simulink model "PhysModel013"  (R2016b)
settings: Solver=VariableStepAuto  StartTime=0.0  StopTime=10.0  RelTol=1e-3
libraries: simulink x2
settings Model: Creator=gwb15193  LastModifiedBy=gwb15193
settings DataIOCC: ReturnWorkspaceOutputs=on
settings SFSimCC: SimUseLocalCustomCode=on
settings RTWCC: RTWUseLocalCustomCode=on

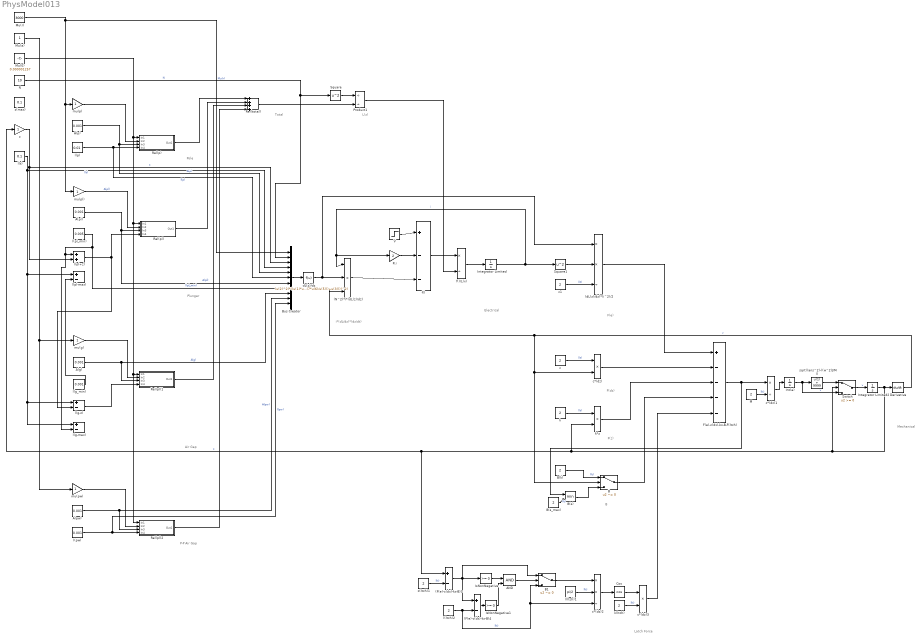
== system PhysModel013 ==
  note: Latch Force
  note: F(dz)
  note: F(e)
  note: i*(dL/dz)*(dz/dt)
  note: Mechanical
  note: Electrical
  note: Total
  note: Pole
  note: Plunger
  note: Air Gap
  note: P-P Air Gap
  note: L(z)
  note: F(z)
  note: B
  (F(e)-c(dx)-kx-B)3 : Sum  Inputs=+-
  (F(e)-c(dx)-kx-B)4 : Sum  Inputs=+-
  (N^2)*i*(dL(z)/dz) : Product  Inputs=***
  (dL(z)/dz)*(i^2)/2 : Product  Inputs=**/
  A(g) : Constant  Value=0.001
  A(p) : Constant  Value=0.001
  A(pl) : Constant  Value=0.001
  A(pw) : Constant  Value=0.001
  AND : Logic  IconShape=distinctive  AllPortsSameDT=off  OutDataTypeStr=boolean
  B : Switch  Criteria=u2 ~= 0
  B(k) : Constant  Value=2
  B(s) : MinMax  Inputs=2
  B(s_max) : Constant  Value=2
  B1 : Switch  Criteria=u2 ~= 0
  Bus Creator : BusCreator  Inputs=11
  Cos : Trigonometry  Operator=cos
  Derivative : Derivative
  F(e)-c(dx)-kx-B-F(ltch) : Sum  Inputs=+----
  Int(a) : Integrator  LimitOutput=on  UpperSaturationLimit=1  LowerSaturationLimit=0
  Integrator Limited : Integrator  LimitOutput=on  UpperSaturationLimit=1  LowerSaturationLimit=0
  Integrator Limited2 : Integrator  LimitOutput=on  UpperSaturationLimit=1  LowerSaturationLimit=0
  IsNonNegative : simulink/Logic and Bit Operations/Compare To Zero  relop=>=  OutDataTypeStr=boolean
  IsNonNegative1 : simulink/Logic and Bit Operations/Compare To Zero  relop=>=  OutDataTypeStr=boolean
  M : Constant  Value=2
  Mu(0) : Constant  Value=0.000001257
  Mu(a) : Constant
  Mu(r) : Constant  Value=3000
  N : Constant  Value=10
  Product1 : Product  Inputs=//
  R.i : Gain  Gain=2
  Rel(p) : Subsystem
  Rel(pl) : Subsystem
  Rel(pl)1 : Subsystem
  Rel(pl)2 : Subsystem
  Rel(total) : Sum  Inputs=++++
  Square : Math  Operator=square  SaturateOnIntegerOverflow=on
  Square1 : Math  Operator=square  SaturateOnIntegerOverflow=on
  Switch : Switch
  V : Step  Time=10  After=10  SampleTime=0
  c : Constant  Value=2
  c*(dz) : Product  Inputs=**
  c*(dz)1 : Product  Inputs=*/
  c*(dz)2 : Product  Inputs=**/
  c*(dz)3 : Product  Inputs=**
  c1 : Constant  Value=2
  dL(z)/dz : Fcn  Expr=(u(2)^2)*((u(1)*u(7)*u(9))*(u(1)*u(7)-u(9))/(((u(1)*u(7))*(u(4)-u(8)+(u(9)*u(11)/u(10))-u(3)))+(u(9)*(u(8)+(u(7*u(6)/u(5)))+u(3))))^2)
  f() : Sum  Inputs=+--
  f()/L(x) : Product  Inputs=*/
  k : Constant  Value=2
  k(ltch) : Constant  Value=2
  k*z : Product  Inputs=**
  l(g-max) : Sum  Inputs=+-
  l(g-z) : Sum  Inputs=+-
  l(g_min) : Constant  Value=0.001
  l(ltch)1 : Constant  Value=pi/2
  l(ltch)2 : Constant  Value=2
  l(p) : Constant  Value=0.01
  l(pl+z) : Sum
  l(pl-max) : Sum  Inputs=+-
  l(pl_min) : Constant  Value=0.005
  l(pw) : Constant  Value=0.001
  l(t) : Constant  Value=0.1
  mu(g) : Gain
  mu(p) : Gain
  mu(pl) : Gain
  mu(pw) : Gain
  sqrt((ans^2)-((w^2)J/M)) : Fcn  Expr=u(1) + 9999
  z : Gain
  z(ltch)1 : Constant  Value=2
  z(max) : Constant  Value=0.1
  wires:
  l(p)/1 -> Bus Creator/6, Rel(p)/4(In4)  "l(p)"
  A(p)/1 -> Bus Creator/5, Rel(p)/3(In3)  "A(p)"
  l(pl+z)/1 -> l(g-z)/2, Rel(pl)/4(In4)
  A(pl)/1 -> Rel(pl)/3(In3), Bus Creator/7  "A(pl)"
  mu(p)/1 -> Rel(p)/2(In2)
  mu(g)/1 -> Rel(pl)1/2(In2)
  A(g)/1 -> Bus Creator/9, Rel(pl)1/3(In3)  "A(g)"
  l(g-z)/1 -> Rel(pl)1/4(In4)
  l(g_min)/1 -> l(pl-max)/2
  A(pw)/1 -> Bus Creator/10, Rel(pl)2/3(In3)  "A(pw)"
  Mu(r)/1 -> Bus Creator/1, mu(pl)/1, mu(p)/1  "Mu(r)"
  l(pw)/1 -> Bus Creator/11, Rel(pl)2/4(In4)  "l(pw)"
  mu(pw)/1 -> Rel(pl)2/2(In2)
  Mu(0)/1 -> Rel(pl)2/1(In1), Rel(pl)1/1(In1), Rel(pl)/1(In1), Rel(p)/1(In1)
  Rel(p)/1(Out1) -> Rel(total)/1
  Rel(pl)/1(Out1) -> Rel(total)/2
  Rel(pl)1/1(Out1) -> Rel(total)/3
  Rel(pl)2/1(Out1) -> Rel(total)/4
  Mu(a)/1 -> mu(pw)/1, mu(g)/1
  l(pl_min)/1 -> Bus Creator/8, l(g-max)/2, l(pl+z)/1  "l(pl_min)"
  z/1 -> l(pl+z)/2, Bus Creator/3  "z"
  Square/1 -> Product1/1
  N/1 -> Bus Creator/2, Square/1  "N"
  Rel(total)/1 -> Product1/2
  f()/L(x)/1 -> Integrator Limited/1
  R.i/1 -> f()/2
  V/1 -> f()/1
  f()/1 -> f()/L(x)/1
  (N^2)*i*(dL(z)/dz)/1 -> f()/3
  Product1/1 -> f()/L(x)/2
  sqrt((ans^2)-((w^2)J/M))/1 -> Switch/1
  Switch/1 -> Integrator Limited2/1  "v"
  Integrator Limited/1 -> R.i/1, (N^2)*i*(dL(z)/dz)/1, Square1/1  "i"
  Int(a)/1 -> sqrt((ans^2)-((w^2)J/M))/1, Switch/3  "v"
  Derivative/1 -> (N^2)*i*(dL(z)/dz)/3, B/2, c*(dz)/2  "v"
  l(t)/1 -> l(g-max)/1, l(g-z)/1, l(pl-max)/1, Bus Creator/4  "l(t)"
  Bus Creator/1 -> dL(z)/dz/1
  dL(z)/dz/1 -> (N^2)*i*(dL(z)/dz)/2, (dL(z)/dz)*(i^2)/2/1
  mu(pl)/1 -> Rel(pl)/2(In2)  "A(pl)"
  c1/1 -> (dL(z)/dz)*(i^2)/2/3  "l(t)"
  Square1/1 -> (dL(z)/dz)*(i^2)/2/2
  (dL(z)/dz)*(i^2)/2/1 -> F(e)-c(dx)-kx-B-F(ltch)/1
  c/1 -> c*(dz)/1  "l(t)"
  c*(dz)/1 -> F(e)-c(dx)-kx-B-F(ltch)/2
  k/1 -> k*z/1  "l(t)"
  k*z/1 -> F(e)-c(dx)-kx-B-F(ltch)/3
  Integrator Limited2/1 -> Switch/2, (F(e)-c(dx)-kx-B)3/1, z/1, k*z/2, Derivative/1  "z"
  B(k)/1 -> B/1  "l(t)"
  B/1 -> F(e)-c(dx)-kx-B-F(ltch)/4
  B(s_max)/1 -> B(s)/2  "l(t)"
  F(e)-c(dx)-kx-B-F(ltch)/1 -> c*(dz)1/1, B(s)/1
  B(s)/1 -> B/3
  c*(dz)1/1 -> Int(a)/1
  M/1 -> c*(dz)1/2  "l(t)"
  l(ltch)2/1 -> B1/3, c*(dz)2/3, (F(e)-c(dx)-kx-B)4/2  "l(t)"
  B1/1 -> c*(dz)2/1
  l(ltch)1/1 -> c*(dz)2/2  "l(t)"
  c*(dz)2/1 -> Cos/1
  Cos/1 -> c*(dz)3/1
  k(ltch)/1 -> c*(dz)3/2  "l(t)"
  z(ltch)1/1 -> (F(e)-c(dx)-kx-B)3/2  "l(t)"
  (F(e)-c(dx)-kx-B)3/1 -> (F(e)-c(dx)-kx-B)4/1, IsNonNegative/1, B1/1
  (F(e)-c(dx)-kx-B)4/1 -> IsNonNegative1/1
  IsNonNegative/1 -> AND/1
  IsNonNegative1/1 -> AND/2
  AND/1 -> B1/2
  c*(dz)3/1 -> F(e)-c(dx)-kx-B-F(ltch)/5

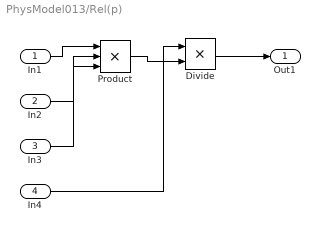
== system PhysModel013/Rel(p) ==
  In1 : Inport
  In2 : Inport  Port=2
  In3 : Inport  Port=3
  In4 : Inport  Port=4
  Divide : Product
  Product : Product  Inputs=3
  Out1 : Outport
  wires:
  In1/1 -> Product/1
  In2/1 -> Product/2
  In3/1 -> Product/3
  In4/1 -> Divide/1
  Product/1 -> Divide/2
  Divide/1 -> Out1/1

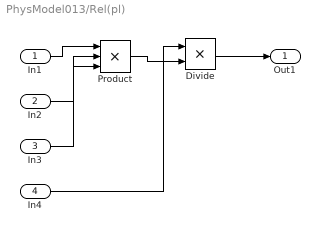
== system PhysModel013/Rel(pl) ==
  In1 : Inport
  In2 : Inport  Port=2
  In3 : Inport  Port=3
  In4 : Inport  Port=4
  Divide : Product
  Product : Product  Inputs=3
  Out1 : Outport
  wires:
  In1/1 -> Product/1
  In2/1 -> Product/2
  In3/1 -> Product/3
  In4/1 -> Divide/1
  Product/1 -> Divide/2
  Divide/1 -> Out1/1

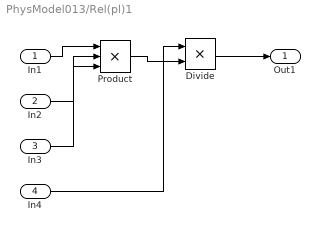
== system PhysModel013/Rel(pl)1 ==
  In1 : Inport
  In2 : Inport  Port=2
  In3 : Inport  Port=3
  In4 : Inport  Port=4
  Divide : Product
  Product : Product  Inputs=3
  Out1 : Outport
  wires:
  In1/1 -> Product/1
  In2/1 -> Product/2
  In3/1 -> Product/3
  In4/1 -> Divide/1
  Product/1 -> Divide/2
  Divide/1 -> Out1/1

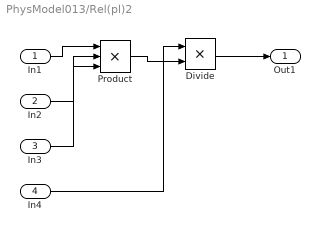
== system PhysModel013/Rel(pl)2 ==
  In1 : Inport
  In2 : Inport  Port=2
  In3 : Inport  Port=3
  In4 : Inport  Port=4
  Divide : Product
  Product : Product  Inputs=3
  Out1 : Outport
  wires:
  In1/1 -> Product/1
  In2/1 -> Product/2
  In3/1 -> Product/3
  In4/1 -> Divide/1
  Product/1 -> Divide/2
  Divide/1 -> Out1/1
